simulink model "stateSpace_design_realtime"  (R2022b)
settings: Solver=VariableStepAuto  StartTime=0.0  StopTime=10.0  RelTol=1e-3
values from neighbouring files (symbols this model uses):
  d = 1/sqrt(2)    [parameters.m]
  K = lqr(sysG, Q, R)    [LQR_Bryson.m]    (also in LQR_design.m; stateSpace_Integral.m = K(2:end); stateSpace_Nominal.m = acker(A,B,eig); stateSpace_design.m = K(2:end))
  Ki = 0    [LQR_Bryson.m]    (also in LQR_design.m; stateSpace_Integral.m = K(1); stateSpace_Nominal.m; stateSpace_design.m = K(1))
  Nu = N(end)    [LQR_Bryson.m]    (also in stateSpace_Integral.m; stateSpace_Nominal.m; stateSpace_design.m)
  Nx = N(1:4)    [LQR_Bryson.m]    (also in stateSpace_Integral.m; stateSpace_Nominal.m; stateSpace_design.m)
  omega_c = 2*pi*50    (= 314.159265359)    [parameters.m]
  rads2rpm = 60/2/pi    (= 9.54929658551)    [parameters.m]
  rpm2rads = 2*pi/60    (= 0.10471975512)    [parameters.m]
undefined symbols (not defined in the file or in its folder): DiscIntNeverNeededParam, National_Instruments, PCIe, sens
libraries: sldrtlib x3, hdlsllib x1
settings Model: Creator=lucas  LastModifiedBy=lucas

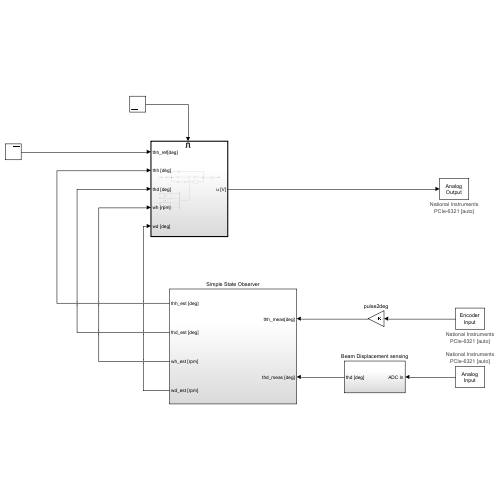
[thumbnail: Simulink's stored preview of the top-level diagram]
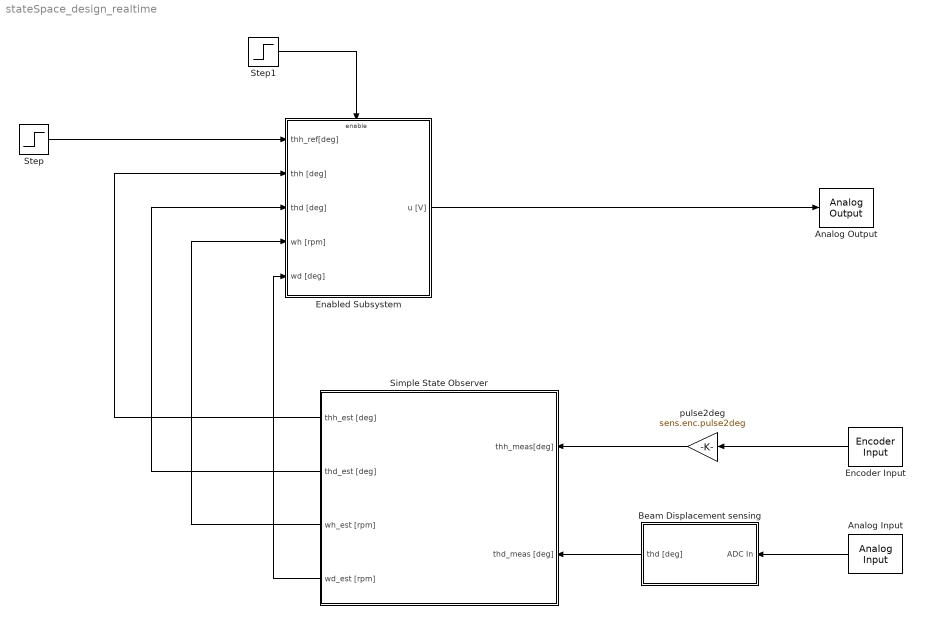
== system stateSpace_design_realtime ==
  Analog Input : sldrtlib/Analog Input  SampleTime=-1  MaxMissedTicks=10  ShowMissedTicks=off  YieldWhenWaiting=off  DrvName=National_Instruments/PCIe-6321  DrvAddress=4294967295  DrvOptions=[0 0 0 2 0 0 0]  Channels=[1, 2]  RangeMode=1  VoltRange=1  DataType=1
      settings: AttributesFormatString=National Instruments\nPCIe-6321 [auto]
  Analog Output : sldrtlib/Analog Output  SampleTime=-1  MaxMissedTicks=10  ShowMissedTicks=off  YieldWhenWaiting=off  DrvName=National_Instruments/PCIe-6321  DrvAddress=4294967295  DrvOptions=[0 0 0 2 0 0 0]  Channels=1  RangeMode=1  VoltRange=1  InitialValue=0  FinalValue=0
      settings: AttributesFormatString=National Instruments\nPCIe-6321 [auto]
  Beam Displacement sensing : Subsystem
  Enabled Subsystem : Subsystem  TreatAsAtomicUnit=on
  Encoder Input : sldrtlib/Encoder Input  SampleTime=-1  MaxMissedTicks=10  ShowMissedTicks=off  YieldWhenWaiting=off  DrvName=National_Instruments/PCIe-6321  DrvAddress=4294967295  DrvOptions=[0 0 0 2 0 0 0]  Channels=1  QuadMode=3  IndexPulse=1  InputFilter=Inf  DataType=1
      settings: AttributesFormatString=National Instruments\nPCIe-6321 [auto]
  Simple State Observer : Subsystem
  Step : Step  After=50
  Step1 : Step  After=50
  pulse2deg : Gain  Gain=sens.enc.pulse2deg
  wires:
  Step/1 -> Enabled Subsystem/1(thh_ref[deg])
  Enabled Subsystem/1(u [V]) -> Analog Output/1
  Encoder Input/1 -> pulse2deg/1
  pulse2deg/1 -> Simple State Observer/1(thh_meas[deg])
  Beam Displacement sensing/1(thd [deg]) -> Simple State Observer/2(thd_meas [deg])
  Analog Input/1 -> Beam Displacement sensing/1(ADC In)
  Simple State Observer/1(thh_est [deg]) -> Enabled Subsystem/2(thh [deg])
  Simple State Observer/2(thd_est [deg]) -> Enabled Subsystem/3(thd [deg])
  Simple State Observer/3(wh_est [rpm]) -> Enabled Subsystem/4(wh [rpm])
  Simple State Observer/4(wd_est [rpm]) -> Enabled Subsystem/5(wd [deg])
  Step1/1 -> Enabled Subsystem/Enable

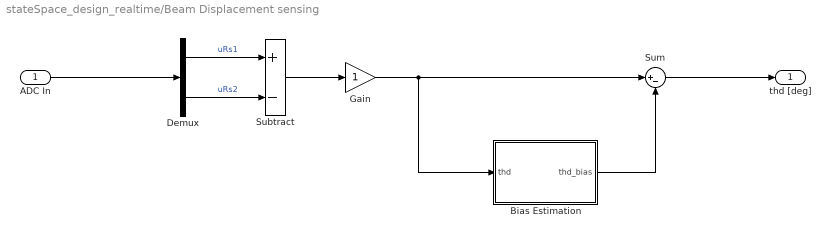
== system stateSpace_design_realtime/Beam Displacement sensing ==
  ADC In : Inport
  Bias Estimation : Subsystem
  Demux : Demux  Outputs=2
  Gain : Gain
  Subtract : Sum  Inputs=+-
  Sum : Sum  Inputs=|+-
  thd [deg] : Outport
  wires:
  Demux/2 -> Subtract/2  "uRs2"
  Demux/1 -> Subtract/1  "uRs1"
  ADC In/1 -> Demux/1
  Subtract/1 -> Gain/1
  Gain/1 -> Bias Estimation/1(thd), Sum/1
  Sum/1 -> thd [deg]/1
  Bias Estimation/1(thd_bias) -> Sum/2

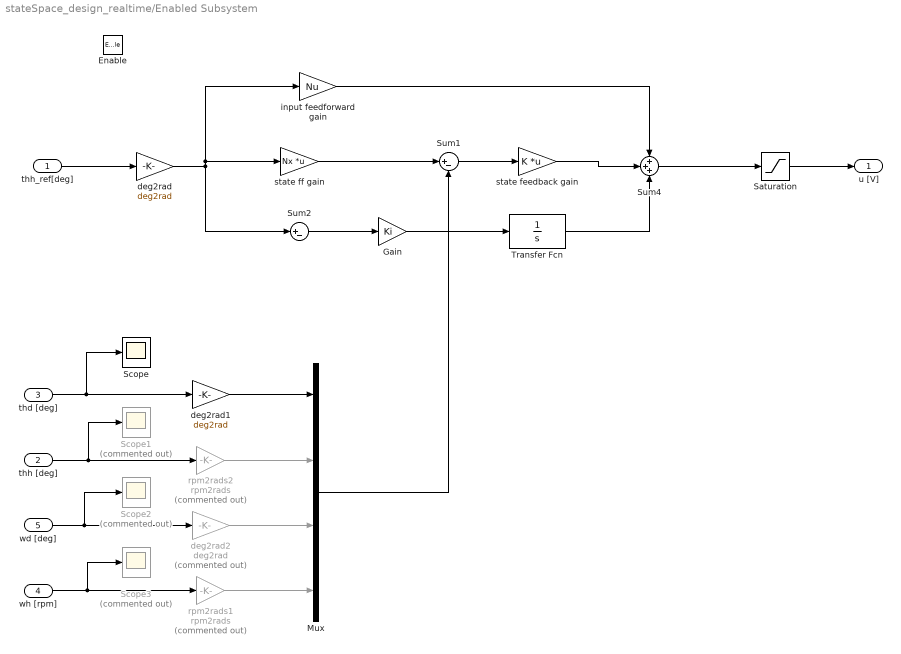
== system stateSpace_design_realtime/Enabled Subsystem ==
  thh_ref[deg] : Inport
  thh [deg] : Inport  Port=2
  thd [deg] : Inport  Port=3
  wh [rpm] : Inport  Port=4
  wd [deg] : Inport  Port=5
  Enable : EnablePort
  " Saturation" : Saturate  UpperLimit=12  LowerLimit=-12
  Gain : Gain  Gain=Ki
  Mux : Mux
  Scope : Scope
  Scope1 : Scope  Commented=on
  Scope2 : Scope  Commented=on
  Scope3 : Scope  Commented=on
  Sum1 : Sum  Inputs=|+-
  Sum2 : Sum  Inputs=|+-
  Sum4 : Sum  Inputs=+++
  Transfer Fcn : TransferFcn  Numerator=1  Denominator=[1 0]
  deg2rad : Gain  Gain=deg2rad
  deg2rad1 : Gain  Gain=deg2rad
  deg2rad2 : Gain  Commented=on  Gain=deg2rad
  input feedforward gain : Gain  Gain=Nu
  rpm2rads1 : Gain  Commented=on  Gain=rpm2rads
  rpm2rads2 : Gain  Commented=on  Gain=rpm2rads
  state feedback gain : Gain  Gain=K  Multiplication=Matrix(K*u) (u vector)
  state ff gain : Gain  Gain=Nx  Multiplication=Matrix(K*u) (u vector)
  u [V] : Outport
  wires:
  deg2rad/1 -> Sum2/1, input feedforward gain/1, state ff gain/1
  thh_ref[deg]/1 -> deg2rad/1
  state ff gain/1 -> Sum1/1
  rpm2rads2/1 -> Mux/2
  Sum1/1 -> state feedback gain/1
  " Saturation"/1 -> u [V]/1
  input feedforward gain/1 -> Sum4/1
  rpm2rads1/1 -> Mux/4
  thh [deg]/1 -> rpm2rads2/1, Scope1/1
  state feedback gain/1 -> Sum4/2
  thd [deg]/1 -> deg2rad1/1, Scope/1
  Mux/1 -> Sum1/2
  deg2rad1/1 -> Mux/1
  Sum4/1 -> " Saturation"/1
  Gain/1 -> Transfer Fcn/1
  Transfer Fcn/1 -> Sum4/3
  deg2rad2/1 -> Mux/3
  wd [deg]/1 -> deg2rad2/1, Scope2/1
  Sum2/1 -> Gain/1
  wh [rpm]/1 -> rpm2rads1/1, Scope3/1

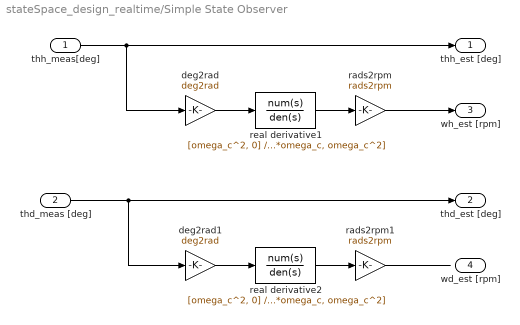
== system stateSpace_design_realtime/Simple State Observer ==
  thh_meas[deg] : Inport
  thd_meas [deg] : Inport  Port=2
  deg2rad : Gain  Gain=deg2rad
  deg2rad1 : Gain  Gain=deg2rad
  rads2rpm : Gain  Gain=rads2rpm
  rads2rpm1 : Gain  Gain=rads2rpm
  real derivative1 : TransferFcn  Numerator=[omega_c^2, 0]  Denominator=[1, 2*d*omega_c, omega_c^2]
  real derivative2 : TransferFcn  Numerator=[omega_c^2, 0]  Denominator=[1, 2*d*omega_c, omega_c^2]
  thh_est [deg] : Outport
  thd_est [deg] : Outport  Port=2
  wh_est [rpm] : Outport  Port=3
  wd_est [rpm] : Outport  Port=4
  wires:
  thh_meas[deg]/1 -> deg2rad/1, thh_est [deg]/1
  thd_meas [deg]/1 -> deg2rad1/1, thd_est [deg]/1
  real derivative1/1 -> rads2rpm/1
  deg2rad/1 -> real derivative1/1
  rads2rpm/1 -> wh_est [rpm]/1
  rads2rpm1/1 -> ?
  deg2rad1/1 -> real derivative2/1
  real derivative2/1 -> rads2rpm1/1

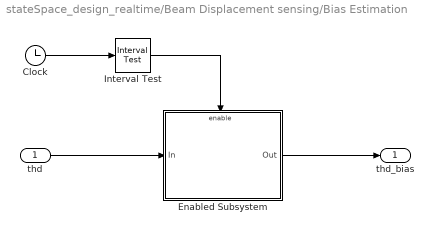
== system stateSpace_design_realtime/Beam Displacement sensing/Bias Estimation ==
  thd : Inport
  Clock : Clock
  Enabled Subsystem : Subsystem  TreatAsAtomicUnit=on
  Interval Test : hdlsllib/Logic and Bit Operations/Interval Test  IntervalClosedRight=on  uplimit=0.5  IntervalClosedLeft=on  lowlimit=-0.5  OutDataTypeStr=boolean
  thd_bias : Outport
  wires:
  thd/1 -> Enabled Subsystem/1(In)
  Enabled Subsystem/1(Out) -> thd_bias/1
  Clock/1 -> Interval Test/1
  Interval Test/1 -> Enabled Subsystem/Enable

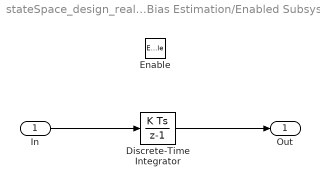
== system stateSpace_design_realtime/Beam Displacement sensing/Bias Estimation/Enabled Subsystem ==
  In : Inport
  Enable : EnablePort
  Discrete-Time Integrator : DiscreteIntegrator  SampleTime=-1  ICPrevOutput=DiscIntNeverNeededParam  ICPrevScaledInput=DiscIntNeverNeededParam
  Out : Outport
  wires:
  In/1 -> Discrete-Time Integrator/1
  Discrete-Time Integrator/1 -> Out/1
